simulink model "exampleCollector1xN"  (R2013b)
settings: Solver=ode45  StartTime=0.0  StopTime=24*3600  RelTol=1e-3
libraries: carnot x6
settings Model: Creator=drhf  LastModifiedBy=drhf
settings DataIOCC: SignalLoggingSaveFormat=ModelDataLogs
settings OptimizationCC: ExpressionDepthLimit=2147483647
settings DebuggingCC: FcnCallInpInsideContextMsg=UseLocalSettings  StateNameClashWarn=warning
settings GRTTargetCC: CombineOutputUpdateFcns=off  GRTInterface=on

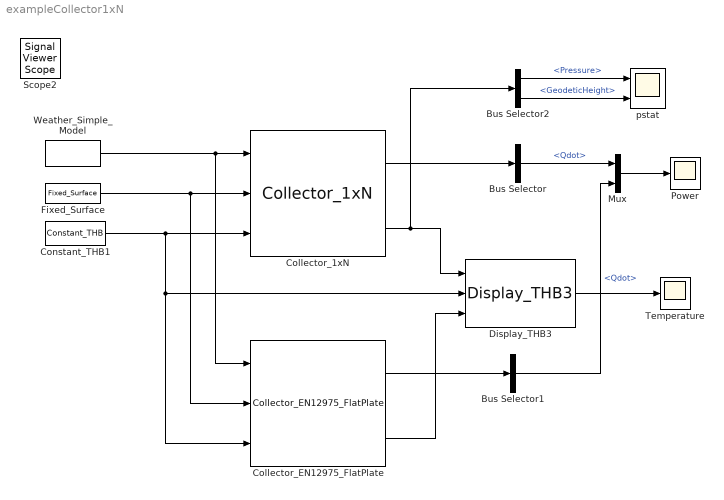
== system exampleCollector1xN ==
  Bus Selector : BusSelector  OutputSignals=Qdot
  Bus Selector1 : BusSelector  OutputSignals=Qdot
  Bus Selector2 : BusSelector  OutputSignals=Pressure,GeodeticHeight
  Collector_1xN : carnot/Source/Solar_Thermal/Collector_1xN  acol=2.3  len=2  eta0=0.8  u1=3.5  u2=0.02  u3=0  uwind=0  c_col=1e4  lin=10  qua=10  tini=20  nodes=5
  Collector_EN12975_FlatPlate : carnot/Source/Solar_Thermal/Collector_EN12975_FlatPlate  acol=2.5  len=2.3  fta=0.8103  c1=3.757  c2=0.0147  c3=0  c4=0  c5=7062  c6=0  b0=0.12  Kd=0.92  lin=0  qua=0  tini=20
  Constant_THB1 : carnot/Source/Simple/Constant_THB  t=40  mdot=100/3600  p=1e5  mID=Full Pressure Drop with Static Height  fluid=Water  mix=0  mix2=0  mix3=0  dia=0.02  hgt=0
  Display_THB3 : carnot/Outputs/Display_THB3  t=on  m=off  p=off  id=off  mix=off  d=off
  Fixed_Surface : carnot/Weather/Fixed_Surface  colangle=30  colazi=0  colrot=0
  Mux : Mux  Inputs=2
  Power : Scope
  Temperature : Scope
  Weather_Simple_Model : carnot/Weather/Weather_Simple_Model  lat=60  Ibn=900  Idg=100  tamb=5  deltaTsky=-6  rh=50  precip="10e-3/24/3600           % 10 mm in 24 h"  cloud=0.125  p=1013e2  vw=1  wdir=270
  pstat : Scope  NumInputPorts=2
      settings: YMin=-5~-5  YMax=5~5  SaveName=ScopeData2
  Scope2 : SignalViewerScope  IOType=viewer  RefreshTime=0.035000
  wires:
  Weather_Simple_Model/1 -> Collector_EN12975_FlatPlate/1, Collector_1xN/1
  Fixed_Surface/1 -> Collector_EN12975_FlatPlate/2, Collector_1xN/2
  Constant_THB1/1 -> Display_THB3/2, Collector_EN12975_FlatPlate/3, Collector_1xN/3
  Collector_1xN/2 -> Display_THB3/1, Bus Selector2/1
  Display_THB3/1 -> Temperature/1
  Collector_EN12975_FlatPlate/2 -> Display_THB3/3
  Collector_1xN/1 -> Bus Selector/1
  Collector_EN12975_FlatPlate/1 -> Bus Selector1/1
  Bus Selector/1 -> Mux/1  "<Qdot>"
  Bus Selector1/1 -> Mux/2  "<Qdot>"
  Mux/1 -> Power/1
  Bus Selector2/1 -> pstat/1  "<Pressure>"
  Bus Selector2/2 -> pstat/2  "<GeodeticHeight>"
